simulink model "cart_simulator"  (R2020a)
settings: Solver=FixedStepAuto  StartTime=0  StopTime=2  FixedStep=0.05  MaxStep=0.02  RelTol=1e-3  AbsTol=1e-6
undefined symbols (not defined in the file): E, pend_length, position_init
Description:
  | Inverted Pendulum with Animation
  | 
  | This example shows how to model an inverted pendulum.  The animation is created using MATLAB(R) Handle Graphics(R).  The animation block is a masked
  | S-function.  For more information, use the context menu to look under the Animation block's mask
  | and open the S-function for editing.
settings Model: EnablePacing=on  ExtModeAutoUpdateStatusClock=off  Creator=The MathWorks, Inc.  LastModifiedBy=yamauchi
settings SolverCC: AutoScaleAbsTol=off
settings DataIOCC: ExternalInput=[]  InitialState=[]  SaveFormat=Array  SaveOutput=off  SaveTime=off
settings OptimizationCC: BlockReduction=off  BooleanDataType=off  ExpressionDepthLimit=2147483647  InitFltsAndDblsToZero=on  LifeSpan=inf
settings DebuggingCC: SaveWithParameterizedLinksMsg=none  UnderspecifiedInitializationDetection=Classic  MergeDetectMultiDrivingBlocksExec=none  SignalResolutionControl=TryResolveAllWithWarning  MultiTaskDSMMsg=warning  MultiTaskCondExecSysMsg=none  SigSpecEnsureSampleTimeMsg=none  FcnCallInpInsideContextMsg=warning  StateNameClashWarn=warning  SFUnexpectedBacktrackingDiag=warning  SFNoUnconditionalDefaultTransitionDiag=warning  SFExecutionAtInitializationDiag=none  ArithmeticOperatorsInVariantConditions=warning
settings HardwareCC: ProdBitPerPointer=32  ProdBitPerSizeT=32  ProdBitPerPtrDiffT=32  ProdLargestAtomicFloat=None  ProdIntDivRoundTo=Undefined  ProdEndianess=Unspecified  ProdWordSize=32  ProdHWDeviceType=32-bit Generic  TargetUnknown=on
settings ModelReferenceCC: PropagateSignalLabelsOutOfModel=off
settings SFSimCC: SimUseLocalCustomCode=off  CustomCodeUndefinedFunction=UseInterfaceOnly
settings RTWCC: RTWUseLocalCustomCode=off
settings CodeAppCC: StateflowObjectComments=on
settings GRTTargetCC: TargetFcnLib=ansi_tfl_tmw.mat  TargetLangStandard=C89/C90 (ANSI)  CombineOutputUpdateFcns=off  GRTInterface=on
settings ConfigComp: CovMetricSettings=dw  CovSaveCumulativeToWorkspaceVar=on  CovSaveSingleToWorkspaceVar=on  CovExternalEMLEnable=off

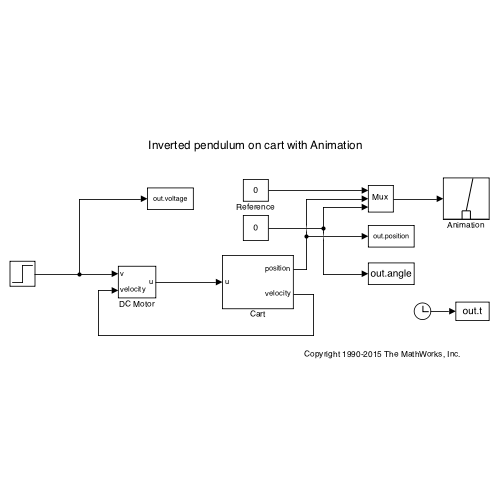
[thumbnail: Simulink's stored preview of the top-level diagram]
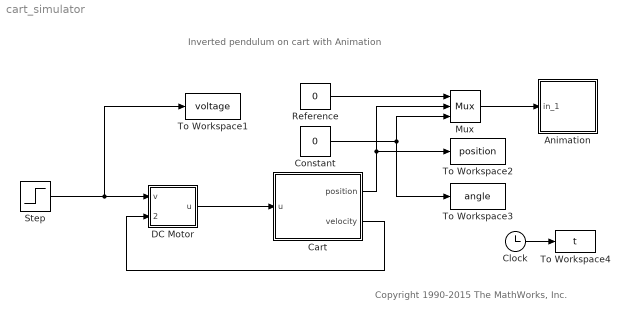
== system cart_simulator ==
  note: Inverted pendulum on cart with Animation
  note: Copyright 1990-2015 The MathWorks, Inc.
  Animation : Subsystem  mask(Pendulum plot){RefBlock=Reference}
      mask prompts: RefBlock "DC reference signal block name:"
      mask help: Pendulum plot
      mask Help: Pendulum animation function using Handle graphics.
      mask Display: plot([-10 10],[0 0],[-2 -2 2 2],[0 1 1 0],[0 3],[1 5])
  Cart : Subsystem  mask(Inverted pendulum on cart){Mcart=0.95, m=0.0568, l=pend_length/2, g=9.8, Dx=1.3, Dt=0.0001}
      mask prompts: Mcart "Mass of cart (kg):"; m "Mass of pendulum (kg):"; l "Distance to pendulum center of mass(m):"; g "Acceleration of gravity (m/s^2):"; Dx "(kg/s)"
      mask help: Unmask and double-click to see dynamics
      mask Help: Nonlinear dynamics of inverted pendulum on cart.
  Clock : Clock
  Constant : Constant  Value=0
  DC Motor : Subsystem  mask(Inverted pendulum on cart){Kg=1, Ke=0.023, rho=0.00635, R=8.3}
      mask prompts: Kg "Gear ratio"; Ke "Back-emf constant (V/(rad/s))"; rho "Radius of pinion gear (m)"; R "Armature resistance (Ohm)"
      mask help: Unmask and double-click to see dynamics
      mask Help: Nonlinear dynamics of inverted pendulum on cart.
  Mux : Mux  Inputs=3
  Reference : Constant  Value=0
  Step : Step  Time=0  After=E  SampleTime=0
  To Workspace1 : ToWorkspace  VariableName=voltage  SampleTime=-1
      settings: Save2DSignal=2-D array (concatenate along first dimension)
  To Workspace2 : ToWorkspace  VariableName=position  SampleTime=-1
      settings: Save2DSignal=2-D array (concatenate along first dimension)
  To Workspace3 : ToWorkspace  VariableName=angle  SampleTime=-1
      settings: Save2DSignal=2-D array (concatenate along first dimension)
  To Workspace4 : ToWorkspace  VariableName=t  SampleTime=-1
      settings: Save2DSignal=2-D array (concatenate along first dimension)
  wires:
  Mux/1 -> Animation/1(in_1)
  Cart/2(velocity) -> DC Motor/2(velocity)
  Cart/1(position) -> To Workspace2/1, Mux/2
  Clock/1 -> To Workspace4/1
  Constant/1 -> To Workspace3/1, Mux/3
  DC Motor/1(u) -> Cart/1(u)
  Step/1 -> To Workspace1/1, DC Motor/1(v)
  Reference/1 -> Mux/1

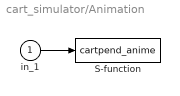
== system cart_simulator/Animation ==
  in_1 : Inport
  S-function : S-Function  FunctionName=cartpend_anime  Parameters=RefBlock  SFunctionDeploymentMode=off  EnableBusSupport=off
      settings: DeleteFcn=pendan([],[],[],'DeleteBlock');
  wires:
  in_1/1 -> S-function/1

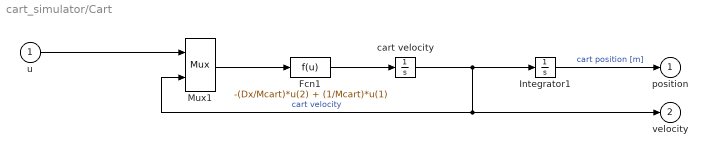
== system cart_simulator/Cart ==
  u : Inport
  Fcn1 : Fcn  Expr=-(Dx/Mcart)*u(2) + (1/Mcart)*u(1)
  Integrator1 : Integrator  InitialCondition=position_init
  Mux1 : Mux  Inputs=2
  cart velocity : Integrator
  position : Outport  InitialOutput=0  VectorParamsAs1DForOutWhenUnconnected=off
  velocity : Outport  Port=2  InitialOutput=0  VectorParamsAs1DForOutWhenUnconnected=off
  wires:
  Integrator1/1 -> position/1  "cart position [m]"
  Fcn1/1 -> cart velocity/1
  cart velocity/1 -> Mux1/2, velocity/1, Integrator1/1  "cart velocity"
  u/1 -> Mux1/1
  Mux1/1 -> Fcn1/1

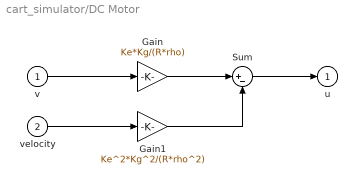
== system cart_simulator/DC Motor ==
  v : Inport
  velocity : Inport  Port=2
  Gain : Gain  Gain=Ke*Kg/(R*rho)
  Gain1 : Gain  Gain=Ke^2*Kg^2/(R*rho^2)
  Sum : Sum  Inputs=|+-
  u : Outport  InitialOutput=0  VectorParamsAs1DForOutWhenUnconnected=off
  wires:
  Sum/1 -> u/1
  v/1 -> Gain/1
  velocity/1 -> Gain1/1
  Gain/1 -> Sum/1
  Gain1/1 -> Sum/2
